simulink model "traj_track_state_error_nonlinear_ctlr"  (R2025b)
settings: Solver=VariableStepAuto  StartTime=0.0  StopTime=10  RelTol=1e-3
libraries: simulink x1, robotmobilelib x1
settings Model: Creator=alessandrochinello  LastModifiedBy=mattc

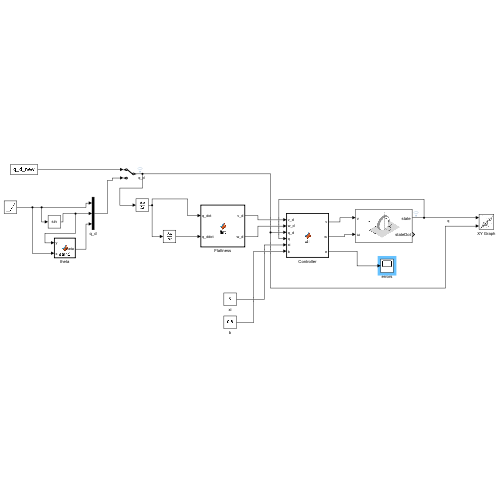
[thumbnail: Simulink's stored preview of the top-level diagram]
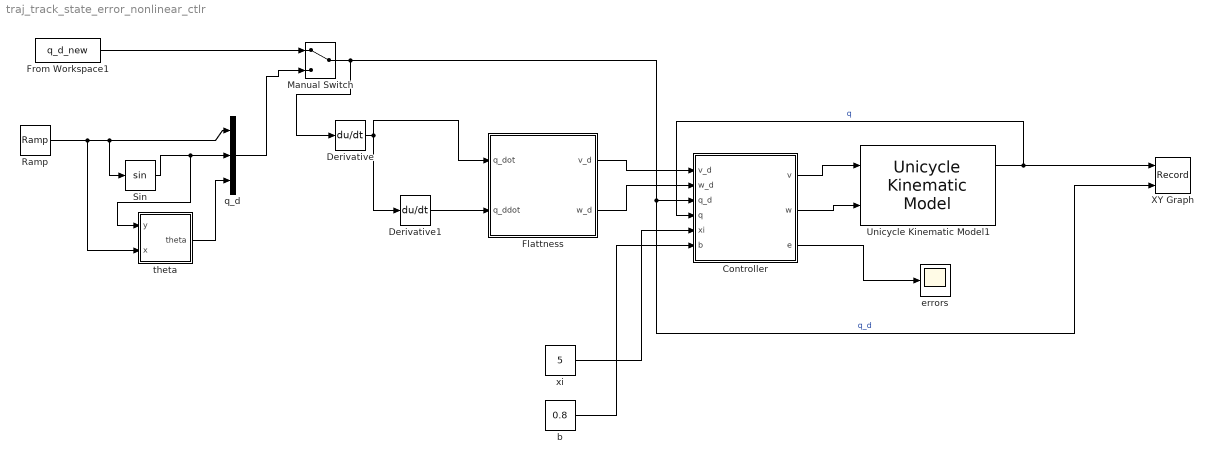
== system traj_track_state_error_nonlinear_ctlr ==
  Controller : MATLAB Function  TreatAsAtomicUnit=on
  Derivative : Derivative
  Derivative1 : Derivative
  Flattness : MATLAB Function  TreatAsAtomicUnit=on
  From Workspace1 : FromWorkspace  VariableName=q_d_new
  Manual Switch : ManualSwitch
  Ramp : simulink/Sources/Ramp  slope=1  start=0  InitialOutput=0
  Sin : Trigonometry
  Unicycle Kinematic Model1 : robotmobilelib/Unicycle Kinematic Model  VehicleInputs=Vehicle Speed & Heading Angular Velocity  WheelRadius=0.1  WheelSpeedRange=[-Inf Inf]  InitialState=q0  SimulateUsing=Interpreted execution
  XY Graph : Record  NumPorts=2.0  FileSettingsInternal="{\"entries\":[{\"content\":{\"excelSettings\":{\"content\":{},\"type\":\"Streamout.ExcelSettings\"},\"parquetSettings\":{\"content\":{},\"type\":\"Streamout.ParquetSettings\"}},\"type\":\"Streamout.FileSettingStorage\",\"uuid\":\"\"}],\"packageUris\":[\"http:\\/\\/schema.mathworks.com\\/mf0\\/streamout_blocks\\/R2020a\"],\"version\":\"1.0\"}"  FrameSettings=[0, 0]  Layout=[1 1]  SignalsInternal="{\"entries\":[{\"content\":{\"signals\":[{\"content\":{\"blockPath\":[],\"dimensions\":[3],\"domain\":\"\",\"hasChildren\":true,\"lineColor\":\"#64d413\",\"lineWidth\":2,\"port\":1,\"sid\":[\"\"],\"signalID\":1,\"signalName\":\"q\"},\"type\":\"RecordBlkView.Signal\",\"uuid\":\"\"},{\"content\":{\"blockPath\":[],\"channel\":[1],\"dimensions\":[3],\"domain\":\"\",\"lineColor\":\"#139fff\",\"lineWidth\":2,\"parentID\":1,\"plots\":[ 1 ],\"port\":1,\"sid\":[\"\"],\"signalID\":2,\"signalName\":\"q\"},\"type\":\"RecordBlkView.Signal\",\"uuid\":\"\"},{\"content\":{\"blockPath\":[],\"dimensions\":[3],\"domain\":\"\",\"hasChildren\":true,\"lineColor\":\"#fe330a\",\"lineWidth\":2,\"port\":2,\"sid\":[\"\"],\"signalID\":3,\"signalName\":\"q_d\"},\"type\":\"RecordBlkView.Signal\",\"uuid\":\"\"},{\"content\":{\"blockPath\":[],\"channel\":[1],\"dimensions\":[3],\"domain\":\"\",\"lineColor\":\"#ff13a6\",\"lineWidth\":2,\"parentID\":3,\"plots\":[ 1 ],\"port\":2,\"sid\":[\"\"],\"signalID\":4,\"signalName\":\"q_d\"},\"type\":\"RecordBlkView.Signal\",\"uuid\":\"\"},{\"content\":{\"blockPath\":[],\"channel\":[2],\"dimensions\":[3],\"domain\":\"\",\"lineColor\":\"#139fff\",\"lineWidth\":2,\"parentID\":1,\"plots\":[ 1 ],\"port\":1,\"sid\":[\"\"],\"signalID\":5,\"signalName\":\"q\"},\"type\":\"RecordBlkView.Signal\",\"uuid\":\"\"},{\"content\":{\"blockPath\":[],\"channel\":[3],\"dimensions\":[3],\"domain\":\"\",\"lineColor\":\"#0072bd\",\"lineWidth\":2,\"parentID\":1,\"port\":1,\"sid\":[\"\"],\"signalID\":6,\"signalName\":\"q\"},\"type\":\"RecordBlkView.Signal\",\"uuid\":\"\"},{\"content\":{\"blockPath\":[],\"channel\":[2],\"dimensions\":[3],\"domain\":\"\",\"lineColor\":\"#ff13a6\",\"lineWidth\":2,\"parentID\":3,\"plots\":[ 1 ],\"port\":2,\"sid\":[\"\"],\"signalID\":7,\"signalName\":\"q_d\"},\"type\":\"RecordBlkView.Signal\",\"uuid\":\"\"},{\"content\":{\"blockPath\":[],\"channel\":[3],\"dimensions\":[3],\"domain\":\"\",\"lineColor\":\"#ff6929\",\"lineWidth\":2,\"parentID\":3,\"port\":2,\"sid\":[\"\"],\"signalID\":8,\"signalName\":\"q_d\"},\"type\":\"RecordBlkView.Signal\",\"uuid\":\"\"}]},\"type\":\"RecordBlkView.InputSignals\",\"uuid\":\"\"}],\"packageUris\":[\"http:\\/\\/schema.mathworks.com\\/mf0\\/streamout_blocks\\/R2020a\"],\"version\":\"1.0\"}"  VisualizationBindings="{\"xyplotplugin\":{\"info\":[{\"series\":[{\"bindingParametersList\":[{\"parameter\":\"X-Axis\",\"signalID\":2,\"signalName\":\"q(1)\"},{\"parameter\":\"Y-Axis\",\"signalID\":5,\"signalName\":\"q(2)\"}],\"seriesID\":0},{\"bindingParametersList\":[{\"parameter\":\"X-Axis\",\"signalID\":4,\"signalName\":\"q_d(1)\"},{\"parameter\":\"Y-Axis\",\"signalID\":7,\"signalName\":\"q_d(2)\"}],\"seriesID\":1}],\"subplotID\":1}]}}"  CompatibilityTag=XY
  b : Constant  Value=0.8
  errors : Scope
      settings: ActiveDisplayYMinimum=-0.80196484104782939  ActiveDisplayYMaximum=0.755474887223013
  q_d : Mux  Inputs=3
  theta : MATLAB Function  TreatAsAtomicUnit=on
  xi : Constant  Value=5
  wires:
  Derivative/1 -> Flattness/1(q_dot), Derivative1/1
  b/1 -> Controller/6(b)
  Unicycle Kinematic Model1/1 -> Controller/4(q), XY Graph/1  "q"
  Manual Switch/1 -> Derivative/1, XY Graph/2, Controller/3(q_d)  "q_d"
  Derivative1/1 -> Flattness/2(q_ddot)
  Controller/3(e) -> errors/1
  Controller/1(v) -> Unicycle Kinematic Model1/1
  Controller/2(w) -> Unicycle Kinematic Model1/2
  Flattness/2(w_d) -> Controller/2(w_d)
  Flattness/1(v_d) -> Controller/1(v_d)
  xi/1 -> Controller/5(xi)
  Sin/1 -> q_d/2, theta/1(y)
  Ramp/1 -> theta/2(x), Sin/1, q_d/1
  theta/1(theta) -> q_d/3
  q_d/1 -> Manual Switch/2
  From Workspace1/1 -> Manual Switch/1

== matlab function traj_track_state_error_nonlinear_ctlr/Controller ==
  data: v_d input; w_d input; q_d input; v output; q input; w output; e output; xi input; b input
function [v, w, e]= ctrl(v_d, w_d, q_d, q, xi, b)

% Get desired state
x_d = q_d(1);
y_d = q_d(2);
theta_d = q_d(3);

% Get (real) theta
x = q(1);
y = q(2);
theta = q(3);

v_d_t = v_d;

% Check if v_d is 0
if abs(v_d) < 1e-4
    if v_d >= 0
        v_d_t = 1e-4;
    else
        v_d_t = -1e-4;
    end
end


k1 = 2*xi*sqrt(b*v_d_t + w_d^2);
k2 = b;
k3 = k1;

% Compute errors
e1 = x_d - x;
e2 = y_d - y;
e3 = theta_d - theta;

v = v_d * cos(e3) + k1 * (e1 * cos(theta) + e2 * sin(theta));
%Check for the singularity, when e3 -> 0
if abs(e3) > 1e-6
    sinc_e3 = sin(e3) / e3;
else
    % taylor aproximation: sin(x)/x approx 1 - x^2/6
    sinc_e3 = 1 - (e3^2) / 6;
end
w = w_d + k2 * (v_d_t * sinc_e3)* (-e1 * sin(theta) + e2 * cos(theta)) + k3 * e3;
e = [e1 e2 e3];

% if isnan(w)
%     disp([v_d_t, k2])
% end

== matlab function traj_track_state_error_nonlinear_ctlr/Flattness ==
  data: q_dot input; q_ddot input; v_d output; w_d output
function [v_d,w_d] = flat(q_dot, q_ddot)

x_dot = q_dot(1);
y_dot = q_dot(2);

x_ddot = q_ddot(1);
y_ddot = q_ddot(2);

norm_2 = x_dot^2 + y_dot^2;

v_d = sqrt(norm_2);
%w_d = q_ddot(3);
if norm_2 <= 1e-4
   w_d = 1e-4;
else
    w_d = (x_dot * y_ddot - x_ddot * y_dot) / (norm_2);
end

== matlab function traj_track_state_error_nonlinear_ctlr/theta ==
  data: y input; x input; theta output
function theta = atan2(y, x)

theta = atan2(y, x);
